simulink model "vrmaglev_statespace"  (R2016b)
settings: Solver=ode5  StartTime=0.0  StopTime=5  FixedStep=1e-3  MaxStep=0.001  RelTol=1e-3  AbsTol=1e-5
model workspace (MATLAB code in the model file):
  | Ts=1e-3;
undefined symbols (not defined in the file): E, H, K, k_follow, L, m, yd
libraries: vrlib x4
Description:
  | Magnetic Levitation Model
  | 
  | vrmaglev is an example showing the interaction between dynamic models in Simulink(R)
  | and virtual worlds. The Simulink model represents the HUMUSOFT(R) CE152 Magnetic Levitation
  | educational / presentation scale model. (http://www.humusoft.com/link/models)
  | 
  | The plant model is controlled by a PID controller with feed forward to cope with the nonlinearity
  | of the magnetic levitation system.
  | 
  | The position of the ball responds to the changing value of the setpoint. You can observe
  | this change not only in the Scope window, but also in a viewer window displaying
  | the virtual world. Note that the position of the ball represents the real dynamics of the system.
  | If you switch the VRML viewer to the Camera 3 viewpoint, you can observe and control the ball easier.
  | 
  | There are two possible methods of setting the ball position setpoint - using a Signal Generator
  | and visually by clicking at a desired position in the virtual reality scene.
  | 
  | In the virtual scene, a VRML sensor is defined. If you click in the space between the magnetic coil
  | and the bottom plate, VRML sensor is updated and its value is read into Simulink model using the
  | VR Source block.
settings Model: FPTRunName=Active  ExtModeTrigDuration=5000  ExtModeTrigLevel=0.500000  Creator=The MathWorks, Inc.  LastModifiedBy=nimaz
settings DataIOCC: SaveFormat=Array  SaveOutput=off  SaveTime=off  SignalLoggingName=logsOut
settings OptimizationCC: BlockReduction=off  BooleanDataType=off  OptimizeBlockIOStorage=off  BufferReuse=off  GlobalBufferReuse=off  ExpressionFolding=off  ExpressionDepthLimit=2147483647  LocalBlockOutputs=off  InitFltsAndDblsToZero=on  LifeSpan=inf
settings DebuggingCC: UnderspecifiedInitializationDetection=Classic  MergeDetectMultiDrivingBlocksExec=none  CheckExecutionContextPreStartOutputMsg=on  SignalResolutionControl=TryResolveAllWithWarning  MultiTaskDSMMsg=warning  MultiTaskCondExecSysMsg=none  FcnCallInpInsideContextMsg=warning  StateNameClashWarn=warning  SFUnexpectedBacktrackingDiag=warning  SFNoUnconditionalDefaultTransitionDiag=warning  SFExecutionAtInitializationDiag=none
settings HardwareCC: ProdBitPerPointer=32  ProdBitPerSizeT=32  ProdBitPerPtrDiffT=32  ProdLargestAtomicFloat=None  ProdIntDivRoundTo=Undefined  ProdEndianess=Unspecified  ProdWordSize=32  ProdHWDeviceType=32-bit Generic  TargetUnknown=on
settings ModelReferenceCC: UpdateModelReferenceTargets=IfOutOfDate  PropagateSignalLabelsOutOfModel=off
settings RTWCC: RetainRTWFile=on
settings GRTTargetCC: TargetFcnLib=ansi_tfl_tmw.mat  TargetLangStandard=C89/C90 (ANSI)  CombineOutputUpdateFcns=off  GRTInterface=on
settings ConfigComp: CovMetricSettings=d  CovSaveCumulativeToWorkspaceVar=on  CovSaveSingleToWorkspaceVar=on  CovExternalEMLEnable=off  CovSFcnEnable=off

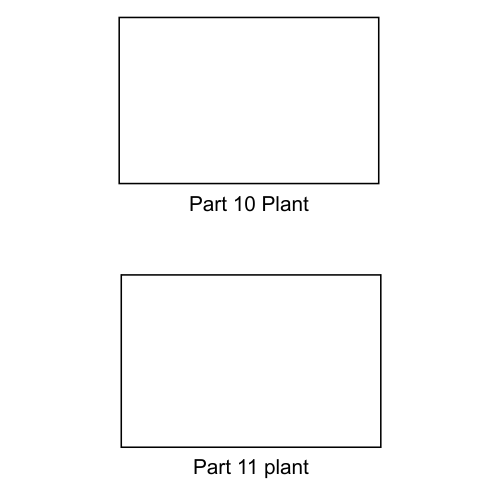
[thumbnail: Simulink's stored preview of the top-level diagram]
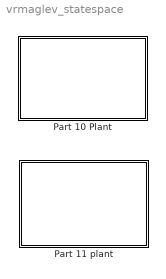
== system vrmaglev_statespace ==
  Part 10 Plant : Subsystem
  Part 11 plant : Subsystem

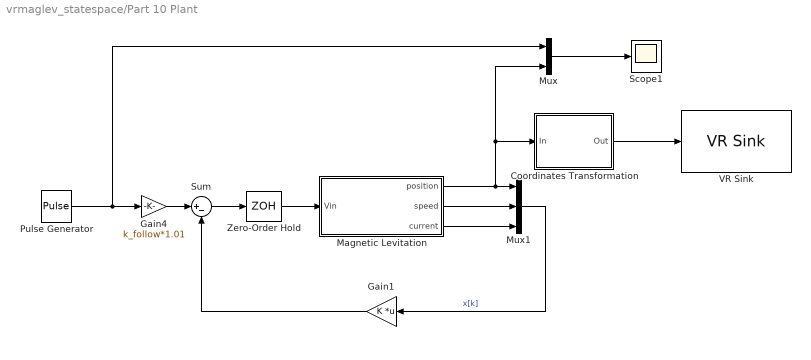
== system vrmaglev_statespace/Part 10 Plant ==
  Coordinates Transformation : Subsystem
  Gain1 : Gain  Gain=K  Multiplication=Matrix(K*u)
  Gain4 : Gain  Gain=k_follow*1.01
  Magnetic Levitation : Subsystem
  Mux : Mux  Inputs=2
  Mux1 : Mux  Inputs=3
  Pulse Generator : DiscretePulseGenerator  PulseType=Time based  Amplitude=yd  Period=11  PulseWidth=50
  Scope1 : Scope
  Sum : Sum  Inputs=|+-  InputSameDT=on  SaturateOnIntegerOverflow=on  OutDataTypeStr=Inherit: Same as first input
  VR Sink : vrlib/VR Sink  InstantiateOnLoad=on  SampleTime=0.02  ViewEnable=on  RemoteChange=off  RemoteView=off  FieldsWritten=Ball.translation.3.1.1.double  WorldFileName=maglev.wrl  WorldDescription=VR Magnetic Levitation Model  AutoView=on  VideoDimensions=[]  AllowVariableSize=off
  Zero-Order Hold : ZeroOrderHold  SampleTime=0.01
  wires:
  Gain1/1 -> Sum/2
  Gain4/1 -> Sum/1
  Coordinates Transformation/1(Out) -> VR Sink/1
  Magnetic Levitation/3(current) -> Mux1/3
  Magnetic Levitation/1(position) -> Mux/2, Coordinates Transformation/1(In), Mux1/1
  Sum/1 -> Zero-Order Hold/1
  Zero-Order Hold/1 -> Magnetic Levitation/1(Vin)
  Pulse Generator/1 -> Mux/1, Gain4/1
  Mux/1 -> Scope1/1
  Magnetic Levitation/2(speed) -> Mux1/2
  Mux1/1 -> Gain1/1  "x[k]"

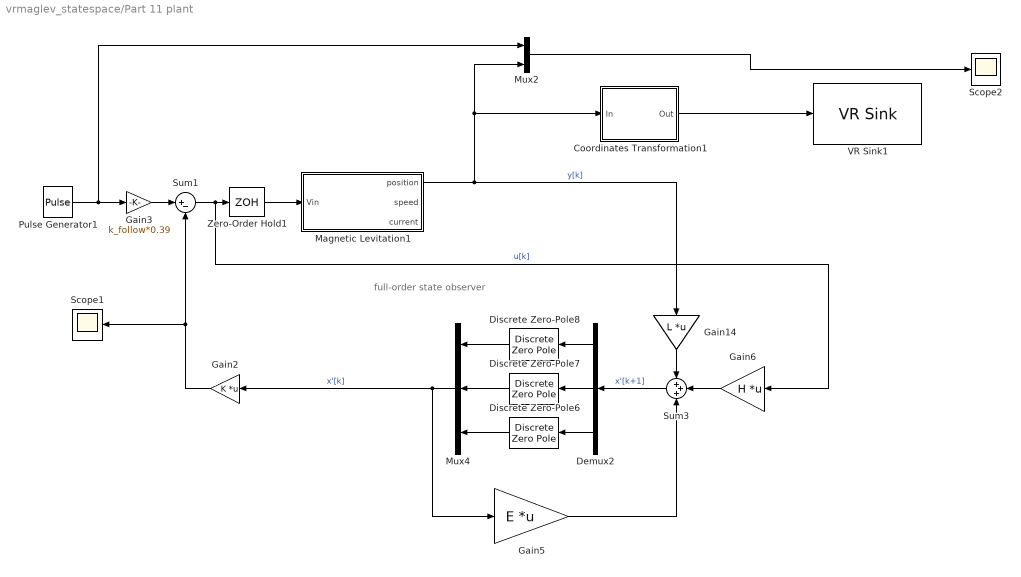
== system vrmaglev_statespace/Part 11 plant ==
  note: full-order state observer
  Coordinates Transformation1 : Subsystem
  Demux2 : Demux  Outputs=3
  Discrete Zero-Pole6 : DiscreteZeroPole  Zeros=[]  Poles=[0]  Gain=1  SampleTime=0.01
  Discrete Zero-Pole7 : DiscreteZeroPole  Zeros=[]  Poles=[0]  Gain=1  SampleTime=0.01
  Discrete Zero-Pole8 : DiscreteZeroPole  Zeros=[]  Poles=[0]  Gain=1  SampleTime=0.01
  Gain14 : Gain  Gain=L  Multiplication=Matrix(K*u)
  Gain2 : Gain  Gain=K  Multiplication=Matrix(K*u)
  Gain3 : Gain  Gain=k_follow*0.39
  Gain5 : Gain  Gain=E  Multiplication=Matrix(K*u)
  Gain6 : Gain  Gain=H  Multiplication=Matrix(K*u)
  Magnetic Levitation1 : Subsystem
  Mux2 : Mux  Inputs=2
  Mux4 : Mux  Inputs=3
  Pulse Generator1 : DiscretePulseGenerator  PulseType=Time based  Amplitude=yd  Period=11  PulseWidth=50
  Scope1 : Scope
  Scope2 : Scope
  Sum1 : Sum  Inputs=|+-  InputSameDT=on  SaturateOnIntegerOverflow=on  OutDataTypeStr=Inherit: Same as first input
  Sum3 : Sum  Inputs=+++
  VR Sink1 : vrlib/VR Sink  InstantiateOnLoad=on  SampleTime=0.02  ViewEnable=on  RemoteChange=off  RemoteView=off  FieldsWritten=Ball.translation.3.1.1.double  WorldFileName=maglev.wrl  WorldDescription=VR Magnetic Levitation Model  AutoView=on  VideoDimensions=[]  AllowVariableSize=off
  Zero-Order Hold1 : ZeroOrderHold  SampleTime=0.01
  wires:
  Discrete Zero-Pole8/1 -> Mux4/1
  Demux2/2 -> Discrete Zero-Pole7/1
  Demux2/3 -> Discrete Zero-Pole6/1
  Discrete Zero-Pole6/1 -> Mux4/3
  Coordinates Transformation1/1(Out) -> VR Sink1/1
  Discrete Zero-Pole7/1 -> Mux4/2
  Gain14/1 -> Sum3/1
  Mux4/1 -> Gain2/1, Gain5/1  "x'[k]"
  Sum3/1 -> Demux2/1  "x'[k+1]"
  Gain6/1 -> Sum3/2
  Gain5/1 -> Sum3/3
  Sum1/1 -> Gain6/1, Zero-Order Hold1/1  "u[k]"
  Pulse Generator1/1 -> Mux2/1, Gain3/1
  Demux2/1 -> Discrete Zero-Pole8/1
  Magnetic Levitation1/1(position) -> Gain14/1, Coordinates Transformation1/1(In), Mux2/2  "y[k]"
  Zero-Order Hold1/1 -> Magnetic Levitation1/1(Vin)
  Gain2/1 -> Scope1/1, Sum1/2
  Gain3/1 -> Sum1/1
  Mux2/1 -> Scope2/1

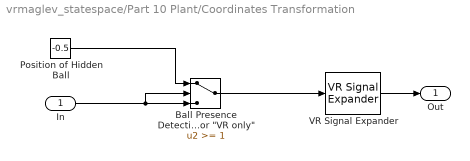
== system vrmaglev_statespace/Part 10 Plant/Coordinates Transformation ==
  In : Inport
  "Ball Presence Detection Value > Threshold = Ball Not Present 1 for \"VR only\"" : Switch  Threshold=1  InputSameDT=on
  Position of Hidden Ball : Constant  Value=-0.5
  VR Signal Expander : vrlib/VR Signal Expander  outwidth=3  outidx=[2]
  Out : Outport
  wires:
  Position of Hidden Ball/1 -> "Ball Presence Detection Value > Threshold = Ball Not Present 1 for \"VR only\""/1
  In/1 -> "Ball Presence Detection Value > Threshold = Ball Not Present 1 for \"VR only\""/3, "Ball Presence Detection Value > Threshold = Ball Not Present 1 for \"VR only\""/2
  "Ball Presence Detection Value > Threshold = Ball Not Present 1 for \"VR only\""/1 -> VR Signal Expander/1
  VR Signal Expander/1 -> Out/1

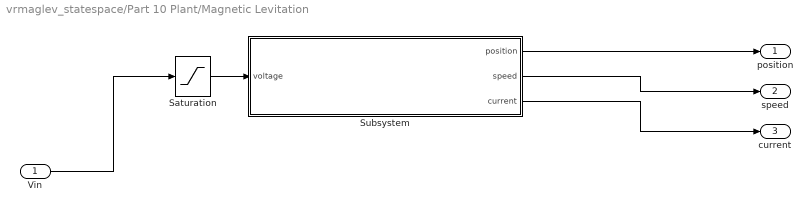
== system vrmaglev_statespace/Part 10 Plant/Magnetic Levitation ==
  Vin : Inport
  Saturation : Saturate  UpperLimit=10  LowerLimit=0  ZeroCross=off
  Subsystem : Subsystem
  position : Outport
  speed : Outport  Port=2
  current : Outport  Port=3
  wires:
  Vin/1 -> Saturation/1
  Saturation/1 -> Subsystem/1(voltage)
  Subsystem/1("position ") -> position/1
  Subsystem/2(speed) -> speed/1
  Subsystem/3(current) -> current/1

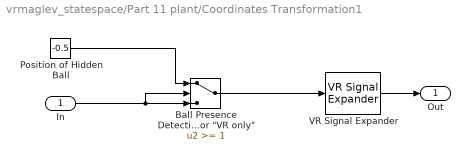
== system vrmaglev_statespace/Part 11 plant/Coordinates Transformation1 ==
  In : Inport
  "Ball Presence Detection Value > Threshold = Ball Not Present 1 for \"VR only\"" : Switch  Threshold=1  InputSameDT=on
  Position of Hidden Ball : Constant  Value=-0.5
  VR Signal Expander : vrlib/VR Signal Expander  outwidth=3  outidx=[2]
  Out : Outport
  wires:
  Position of Hidden Ball/1 -> "Ball Presence Detection Value > Threshold = Ball Not Present 1 for \"VR only\""/1
  In/1 -> "Ball Presence Detection Value > Threshold = Ball Not Present 1 for \"VR only\""/3, "Ball Presence Detection Value > Threshold = Ball Not Present 1 for \"VR only\""/2
  "Ball Presence Detection Value > Threshold = Ball Not Present 1 for \"VR only\""/1 -> VR Signal Expander/1
  VR Signal Expander/1 -> Out/1

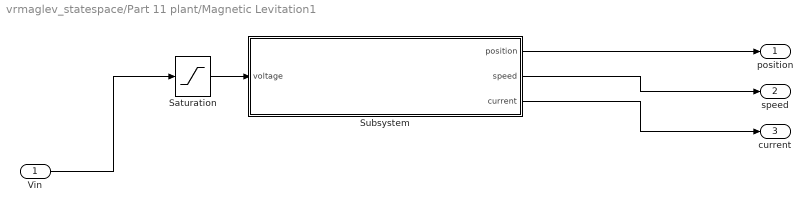
== system vrmaglev_statespace/Part 11 plant/Magnetic Levitation1 ==
  Vin : Inport
  Saturation : Saturate  UpperLimit=10  LowerLimit=0  ZeroCross=off
  Subsystem : Subsystem
  position : Outport
  speed : Outport  Port=2
  current : Outport  Port=3
  wires:
  Vin/1 -> Saturation/1
  Saturation/1 -> Subsystem/1(voltage)
  Subsystem/1("position ") -> position/1
  Subsystem/2(speed) -> speed/1
  Subsystem/3(current) -> current/1

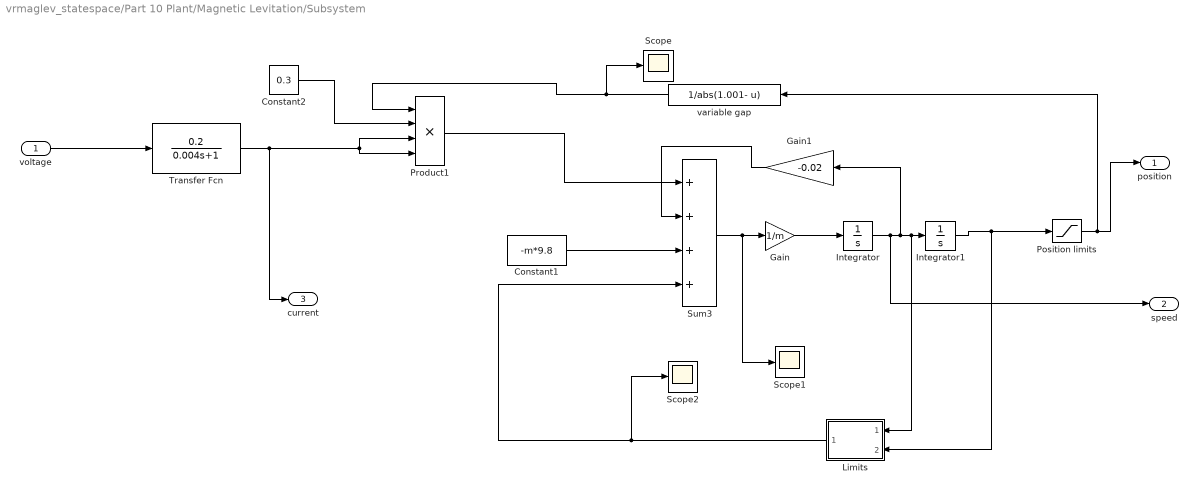
== system vrmaglev_statespace/Part 10 Plant/Magnetic Levitation/Subsystem ==
  voltage : Inport
  Constant1 : Constant  Value=-m*9.8
  Constant2 : Constant  Value=0.3
  Gain : Gain  Gain=1/m
  Gain1 : Gain  Gain=-0.02
  Integrator : Integrator
  Integrator1 : Integrator  LimitOutput=on  UpperSaturationLimit=1  LowerSaturationLimit=0
  Limits : Subsystem
      mask Display: disp('LIMIT')
  Position limits : Saturate  UpperLimit=0.998  LowerLimit=0.001  ZeroCross=off
  Product1 : Product  Inputs=4
  Scope : Scope
  Scope1 : Scope
  Scope2 : Scope
  Sum3 : Sum  Inputs=++++
  Transfer Fcn : TransferFcn  Numerator=[0.2]  Denominator=[0.004 1]
  variable gap : Fcn  Expr=1/abs(1.001- u)
  "position " : Outport
  speed : Outport  Port=2
  current : Outport  Port=3
  wires:
  Position limits/1 -> variable gap/1, "position "/1
  Integrator1/1 -> Limits/2(position), Position limits/1
  Sum3/1 -> Scope1/1, Gain/1
  Constant2/1 -> Product1/2
  Constant1/1 -> Sum3/3
  variable gap/1 -> Scope/1, Product1/1
  Gain1/1 -> Sum3/2
  Gain/1 -> Integrator/1
  Integrator/1 -> speed/1, Limits/1(velocity), Integrator1/1, Gain1/1
  Product1/1 -> Sum3/1
  Transfer Fcn/1 -> current/1, Product1/3, Product1/4
  voltage/1 -> Transfer Fcn/1
  Limits/1(force) -> Scope2/1, Sum3/4

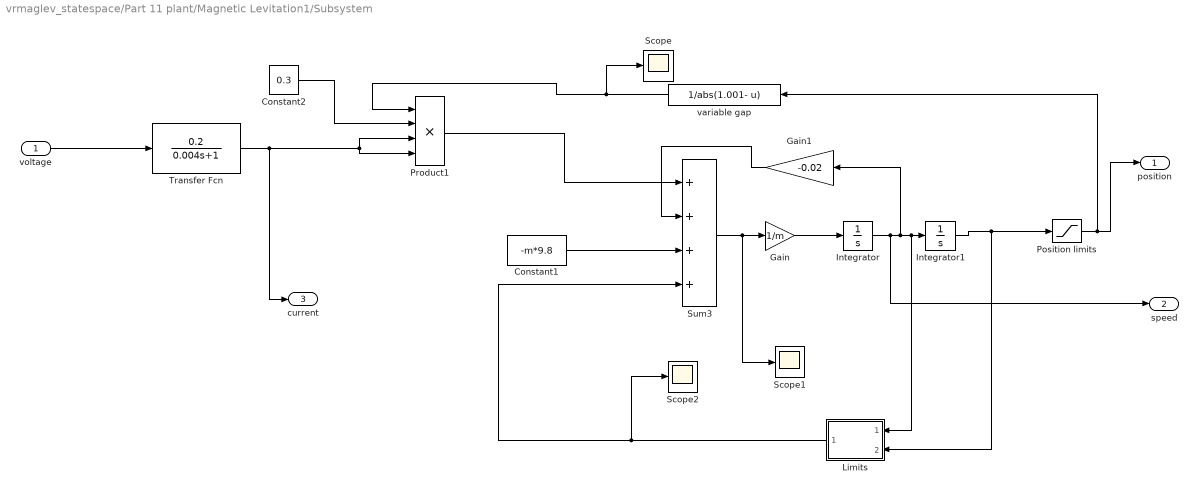
== system vrmaglev_statespace/Part 11 plant/Magnetic Levitation1/Subsystem ==
  voltage : Inport
  Constant1 : Constant  Value=-m*9.8
  Constant2 : Constant  Value=0.3
  Gain : Gain  Gain=1/m
  Gain1 : Gain  Gain=-0.02
  Integrator : Integrator
  Integrator1 : Integrator  LimitOutput=on  UpperSaturationLimit=1  LowerSaturationLimit=0
  Limits : Subsystem
      mask Display: disp('LIMIT')
  Position limits : Saturate  UpperLimit=0.998  LowerLimit=0.001  ZeroCross=off
  Product1 : Product  Inputs=4
  Scope : Scope
  Scope1 : Scope
  Scope2 : Scope
  Sum3 : Sum  Inputs=++++
  Transfer Fcn : TransferFcn  Numerator=[0.2]  Denominator=[0.004 1]
  variable gap : Fcn  Expr=1/abs(1.001- u)
  "position " : Outport
  speed : Outport  Port=2
  current : Outport  Port=3
  wires:
  Position limits/1 -> variable gap/1, "position "/1
  Integrator1/1 -> Limits/2(position), Position limits/1
  Sum3/1 -> Scope1/1, Gain/1
  Constant2/1 -> Product1/2
  Constant1/1 -> Sum3/3
  variable gap/1 -> Scope/1, Product1/1
  Gain1/1 -> Sum3/2
  Gain/1 -> Integrator/1
  Integrator/1 -> speed/1, Limits/1(velocity), Integrator1/1, Gain1/1
  Product1/1 -> Sum3/1
  Transfer Fcn/1 -> current/1, Product1/3, Product1/4
  voltage/1 -> Transfer Fcn/1
  Limits/1(force) -> Scope2/1, Sum3/4

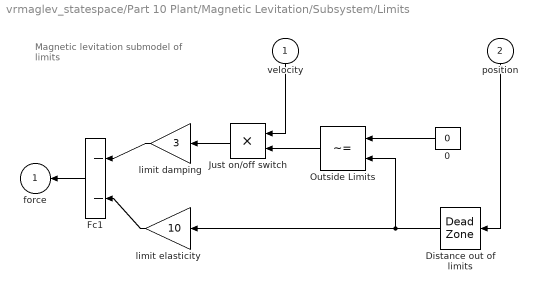
== system vrmaglev_statespace/Part 10 Plant/Magnetic Levitation/Subsystem/Limits ==
  note: Magnetic levitation
      | submodel of limits
  velocity : Inport
  position : Inport  Port=2
  0 : Constant  Value=0
  Distance out of limits : DeadZone  LowerValue=0.002  UpperValue=1  ZeroCross=off  SaturateOnIntegerOverflow=on
  Fc1 : Sum  Inputs=--  InputSameDT=on  SaturateOnIntegerOverflow=on  OutDataTypeStr=Inherit: Same as first input
  "Just on/off switch " : Product  InputSameDT=on  SaturateOnIntegerOverflow=on  OutDataTypeStr=Inherit: Same as first input
  Outside Limits : RelationalOperator  Operator=~=  RndMeth=Nearest  InputSameDT=on
  limit damping : Gain  Gain=3  SaturateOnIntegerOverflow=on  OutDataTypeStr=Inherit: Same as input  ParamDataTypeStr=Inherit: Same as input
  limit elasticity : Gain  Gain=10  SaturateOnIntegerOverflow=on  OutDataTypeStr=Inherit: Same as input  ParamDataTypeStr=Inherit: Same as input
  force : Outport
  wires:
  Distance out of limits/1 -> Outside Limits/2, limit elasticity/1
  limit damping/1 -> Fc1/1
  limit elasticity/1 -> Fc1/2
  Outside Limits/1 -> "Just on/off switch "/2
  0/1 -> Outside Limits/1
  "Just on/off switch "/1 -> limit damping/1
  velocity/1 -> "Just on/off switch "/1
  Fc1/1 -> force/1
  position/1 -> Distance out of limits/1

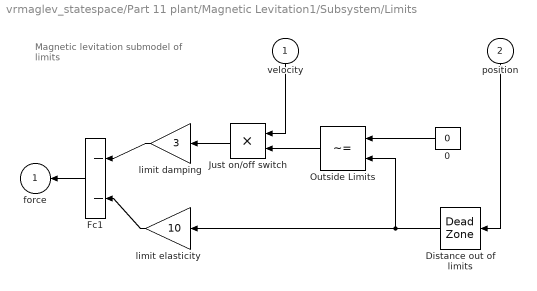
== system vrmaglev_statespace/Part 11 plant/Magnetic Levitation1/Subsystem/Limits ==
  note: Magnetic levitation
      | submodel of limits
  velocity : Inport
  position : Inport  Port=2
  0 : Constant  Value=0
  Distance out of limits : DeadZone  LowerValue=0.002  UpperValue=1  ZeroCross=off  SaturateOnIntegerOverflow=on
  Fc1 : Sum  Inputs=--  InputSameDT=on  SaturateOnIntegerOverflow=on  OutDataTypeStr=Inherit: Same as first input
  "Just on/off switch " : Product  InputSameDT=on  SaturateOnIntegerOverflow=on  OutDataTypeStr=Inherit: Same as first input
  Outside Limits : RelationalOperator  Operator=~=  RndMeth=Nearest  InputSameDT=on
  limit damping : Gain  Gain=3  SaturateOnIntegerOverflow=on  OutDataTypeStr=Inherit: Same as input  ParamDataTypeStr=Inherit: Same as input
  limit elasticity : Gain  Gain=10  SaturateOnIntegerOverflow=on  OutDataTypeStr=Inherit: Same as input  ParamDataTypeStr=Inherit: Same as input
  force : Outport
  wires:
  Distance out of limits/1 -> Outside Limits/2, limit elasticity/1
  limit damping/1 -> Fc1/1
  limit elasticity/1 -> Fc1/2
  Outside Limits/1 -> "Just on/off switch "/2
  0/1 -> Outside Limits/1
  "Just on/off switch "/1 -> limit damping/1
  velocity/1 -> "Just on/off switch "/1
  Fc1/1 -> force/1
  position/1 -> Distance out of limits/1
